simulink model "Start"  (R2016b)
settings: Solver=FixedStepDiscrete  StartTime=0.0  StopTime=60  FixedStep=0.0001  MaxStep=0.001  RelTol=1e-3
undefined symbols (not defined in the file): kat
libraries: simulink x9, microdaq_lib x5
settings Model: SimulationMode=external  ExtModeTrigDuration=10000  Creator=student  LastModifiedBy=barte
settings DataIOCC: MaxDataPoints=100000  SaveFormat=Array
settings DebuggingCC: ParameterTunabilityLossMsg=error
settings HardwareCC: ProdBitPerLong=40  ProdBitPerPointer=32  ProdBitPerSizeT=32  ProdBitPerPtrDiffT=32  ProdLargestAtomicInteger=Integer  ProdLargestAtomicFloat=None  ProdWordSize=32  ProdHWDeviceType=Texas Instruments->C6000
settings RTWCC: SystemTargetFile=microdaq.tlc  TemplateMakefile=microdaq.tmf  PostCodeGenCommand=microdaq_postcodegen(buildInfo)  Description=MicroDAQ Real-Time Measurement System  GenerateReport=on  IncludeHyperlinkInReport=on  LaunchReport=on  GenerateTraceInfo=on  GenerateTraceReport=on  GenerateTraceReportSl=on  GenerateTraceReportSf=on  GenerateTraceReportEml=on
settings CodeAppCC: ForceParamTrailComments=on  IgnoreCustomStorageClasses=off  OperatorAnnotations=on  SimulinkDataObjDesc=on  SFDataObjDesc=on  MATLABFcnDesc=on  InsertBlockDesc=on  MATLABSourceComments=on
settings STFCustomTargetCC: TargetLangStandard=C99 (ISO)  CombineOutputUpdateFcns=on  ERTCustomFileBanners=on  SupportNonInlinedSFcns=off  RemoveResetFunc=on  MATLABClassNameForMDSCustomization=Simulink.SoftwareTarget.ERTCustomization  GRTInterface=off  SystemTargetFile=microdaq.tlc
settings ERTTargetCC: TargetLangStandard=C99 (ISO)  ParMdlRefBuildCompliant=off  CompOptLevelCompliant=off  ConcurrentExecutionCompliant=off  ERTFirstTimeCompliant=off  SupportContinuousTime=on  ModelStepFunctionPrototypeControlCompliant=off  CPPClassGenCompliant=off  UseToolchainInfoCompliant=off  ExtMode=on  ExtModeStaticAlloc=on  ExtModeStaticAllocSize=1085760  ExtModeMexArgs=getpref('microdaq','TargetIP') 1 4344  ERTCustomFileTemplate=microdaq_main.tlc

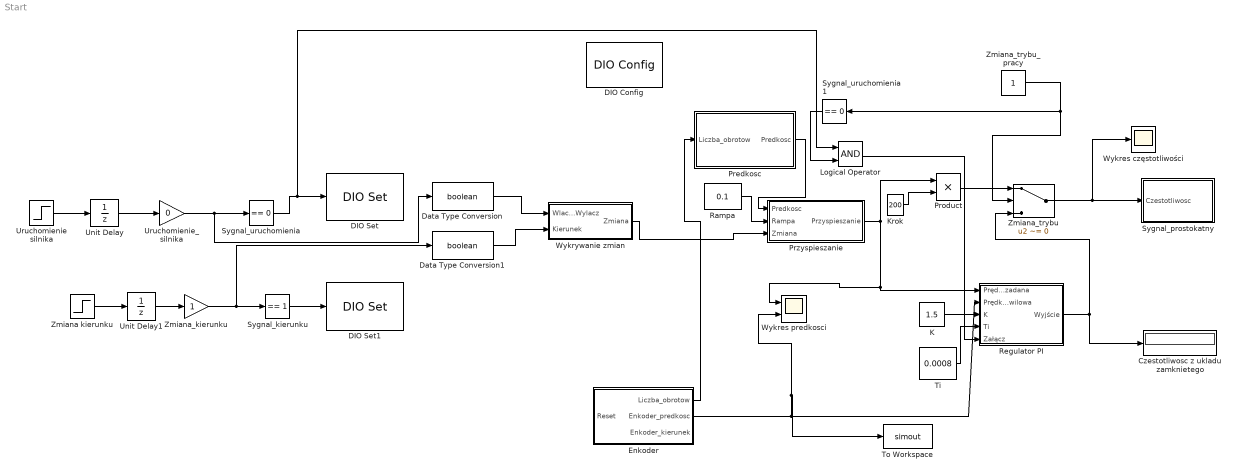
== system Start ==
  "Czestotliwosc z ukladu zamknietego " : Display
  DIO Config : microdaq_lib/Digital/DIO Config  SParameter1=Enable  SParameter2=Enable  SParameter3=Enable  SParameter4=Enable  SParameter5=Enable  SParameter6=Enable  SParameter7=Input  SParameter8=Output  SParameter9=Output  SParameter10=Input
  DIO Set : microdaq_lib/Digital/DIO Set  pDIOpin=DIO21  pDIOdir=ones([1 1 ])  pDIOinitValue=Low  pDIOtermValue=High  SampleTime=-1
  DIO Set1 : microdaq_lib/Digital/DIO Set  pDIOpin=DIO19  pDIOdir=ones([1 1 ])  pDIOinitValue=Low  pDIOtermValue=High  SampleTime=-1
  Data Type Conversion : DataTypeConversion  OutDataTypeStr=boolean
  Data Type Conversion1 : DataTypeConversion  OutDataTypeStr=boolean
  Enkoder : Subsystem
  "K " : Constant  Value=1.5
  "Krok " : Constant  Value=200
  Logical Operator : Logic  AllPortsSameDT=off  OutDataTypeStr=boolean
  Predkosc : Subsystem
  Product : Product  OutDataTypeStr=uint32  RndMeth=Round
  Przyspieszanie : Subsystem
  Rampa : Constant  Value=0.1  OutDataTypeStr=double
  Regulator PI : Subsystem
  Sygnal_kierunku : simulink/Logic and Bit Operations/Compare To Constant  relop===  const=1  OutDataTypeStr=uint8
  Sygnal_prostokatny : Subsystem
  Sygnal_uruchomienia : simulink/Logic and Bit Operations/Compare To Constant  relop===  const=0  OutDataTypeStr=uint8
  Sygnal_uruchomienia1 : simulink/Logic and Bit Operations/Compare To Constant  relop===  const=0  OutDataTypeStr=uint8
  Ti : Constant  Value=0.0008
  To Workspace : ToWorkspace  VariableName=simout  SaveFormat=Timeseries  SampleTime=0.01
  Unit Delay : UnitDelay  SampleTime=-1
  Unit Delay1 : UnitDelay  SampleTime=-1
  Uruchomienie silnika : Step  Time=0.01  SampleTime=0.01
  Uruchomienie_silnika : Gain  Gain=0
  Wykres częstotliwości : Scope
  Wykres predkosci : Scope  NumInputPorts=2
  Wykrywanie zmian : Subsystem
  Zmiana kierunku : Step  Time=0.01  SampleTime=0.01
  Zmiana_kierunku : Gain
  Zmiana_trybu : Switch  Criteria=u2 ~= 0
  Zmiana_trybu_pracy : Constant
  wires:
  Wykrywanie zmian/1(Zmiana) -> Przyspieszanie/3(Zmiana)
  "Krok "/1 -> Product/2
  Rampa/1 -> Przyspieszanie/2(Rampa)
  Data Type Conversion1/1 -> Wykrywanie zmian/2(Kierunek)
  Zmiana kierunku/1 -> Unit Delay1/1
  Uruchomienie silnika/1 -> Unit Delay/1
  Sygnal_kierunku/1 -> DIO Set1/1
  Sygnal_uruchomienia/1 -> Logical Operator/1, DIO Set/1
  Unit Delay/1 -> Uruchomienie_silnika/1
  Unit Delay1/1 -> Zmiana_kierunku/1
  "K "/1 -> Regulator PI/3(K)
  Ti/1 -> Regulator PI/4(Ti)
  Uruchomienie_silnika/1 -> Sygnal_uruchomienia/1, Data Type Conversion/1
  Zmiana_trybu_pracy/1 -> Sygnal_uruchomienia1/1, Zmiana_trybu/2
  Regulator PI/1(Wyjście) -> "Czestotliwosc z ukladu zamknietego "/1, Zmiana_trybu/3
  Zmiana_kierunku/1 -> Data Type Conversion1/1, Sygnal_kierunku/1
  Zmiana_trybu/1 -> Wykres częstotliwości/1, Sygnal_prostokatny/1(Czestotliwosc)
  Przyspieszanie/1(Przyspieszanie) -> Wykres predkosci/1, Regulator PI/1(Prędkość zadana), Product/1
  Product/1 -> Zmiana_trybu/1
  Predkosc/1(Predkosc) -> Przyspieszanie/1(Predkosc)
  Enkoder/1(Liczba_obrotow) -> Predkosc/1(Liczba_obrotow)
  Enkoder/2(Enkoder_predkosc) -> To Workspace/1, Wykres predkosci/2, Regulator PI/2(Prędkość chwilowa)
  Data Type Conversion/1 -> Wykrywanie zmian/1(Wlacz/Wylacz)
  Sygnal_uruchomienia1/1 -> Logical Operator/2
  Logical Operator/1 -> Regulator PI/5(Załącz)

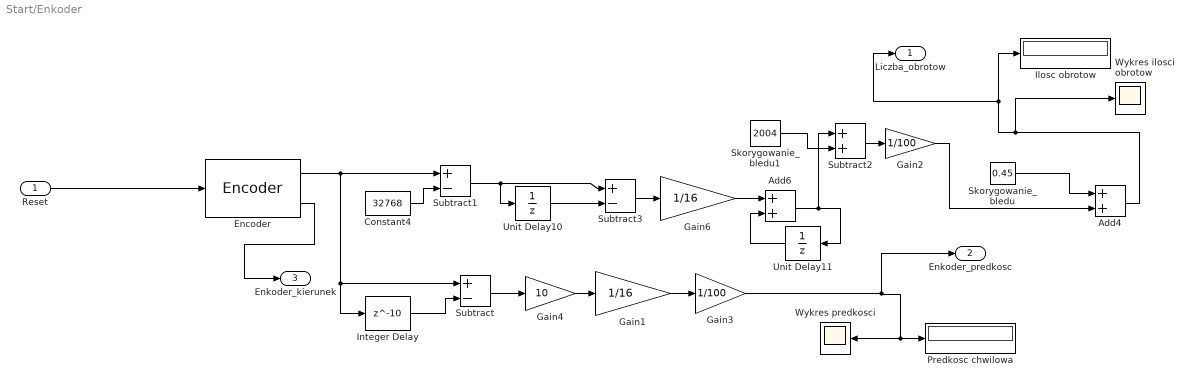
== system Start/Enkoder ==
  Reset : Inport
  Add4 : Sum
  Add6 : Sum  OutDataTypeStr=int32
  Constant4 : Constant  Value=32768  OutDataTypeStr=uint16
  Encoder : microdaq_lib/Motor Control/Encoder  pChannel=ENC1  SampleTime=0.01
  Gain1 : Gain  Gain=1/16  ParamDataTypeStr=double  OutDataTypeStr=int16  RndMeth=Round
  Gain2 : Gain  Gain=1/100
  Gain3 : Gain  Gain=1/100  ParamDataTypeStr=double  OutDataTypeStr=int16  RndMeth=Round
  Gain4 : Gain  Gain=10  ParamDataTypeStr=double  OutDataTypeStr=int16  RndMeth=Round
  Gain6 : Gain  Gain=1/16  ParamDataTypeStr=double  OutDataTypeStr=int16  RndMeth=Round
  "Ilosc obrotow " : Display
      settings: Decimation=2
  Integer Delay : Delay  DelayLength=10
  "Predkosc chwilowa " : Display
      settings: Decimation=2
  Skorygowanie_bledu : Constant  Value=0.45  OutDataTypeStr=double
  Skorygowanie_bledu1 : Constant  Value=2004
  Subtract : Sum  Inputs=+-  AccumDataTypeStr=int16  OutDataTypeStr=uint16  RndMeth=Round
  Subtract1 : Sum  Inputs=+-  OutDataTypeStr=int16
  Subtract2 : Sum  OutDataTypeStr=int16
  Subtract3 : Sum  Inputs=+-  OutDataTypeStr=int16
  Unit Delay10 : UnitDelay  SampleTime=0.01
  Unit Delay11 : UnitDelay  SampleTime=0.01
  "Wykres ilosci obrotow " : Scope
  Wykres predkosci : Scope
  Liczba_obrotow : Outport
  Enkoder_predkosc : Outport  Port=2
  Enkoder_kierunek : Outport  Port=3
  wires:
  Encoder/2 -> Enkoder_kierunek/1
  Reset/1 -> Encoder/1
  Encoder/1 -> Subtract/1, Integer Delay/1, Subtract1/1
  Unit Delay11/1 -> Add6/2
  Unit Delay10/1 -> Subtract3/2
  Subtract3/1 -> Gain6/1
  Integer Delay/1 -> Subtract/2
  Constant4/1 -> Subtract1/2
  Gain6/1 -> Add6/1
  Subtract1/1 -> Subtract3/1, Unit Delay10/1
  Skorygowanie_bledu1/1 -> Subtract2/2
  Add6/1 -> Unit Delay11/1, Subtract2/1
  Subtract2/1 -> Gain2/1
  Skorygowanie_bledu/1 -> Add4/1
  Gain2/1 -> Add4/2
  Add4/1 -> Liczba_obrotow/1, "Ilosc obrotow "/1, "Wykres ilosci obrotow "/1
  Gain1/1 -> Gain3/1
  Subtract/1 -> Gain4/1
  Gain3/1 -> Enkoder_predkosc/1, "Predkosc chwilowa "/1, Wykres predkosci/1
  Gain4/1 -> Gain1/1

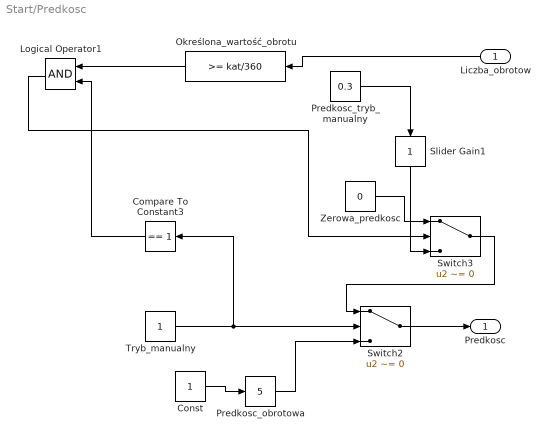
== system Start/Predkosc ==
  Liczba_obrotow : Inport
  Compare To Constant3 : simulink/Logic and Bit Operations/Compare To Constant  relop===  const=1  OutDataTypeStr=uint8
  Const : Constant
  Logical Operator1 : Logic  AllPortsSameDT=off  OutDataTypeStr=boolean
  Określona_wartość_obrotu : simulink/Logic and Bit Operations/Compare To Constant  relop=>=  const=kat/360  OutDataTypeStr=uint8
  Predkosc_obrotowa : simulink/Math Operations/Slider Gain  low=0  gain=5  high=10
  Predkosc_tryb_manualny : Constant  Value=0.3
  Slider Gain1 : simulink/Math Operations/Slider Gain  low=0  gain=1  high=1
  Switch2 : Switch  Criteria=u2 ~= 0  Threshold=1  OutDataTypeStr=double
  Switch3 : Switch  Criteria=u2 ~= 0  Threshold=1  OutDataTypeStr=double
  Tryb_manualny : Constant
  Zerowa_predkosc : Constant  Value=0
  Predkosc : Outport
  wires:
  Slider Gain1/1 -> Switch3/3
  Predkosc_tryb_manualny/1 -> Slider Gain1/1
  Tryb_manualny/1 -> Switch2/2, Compare To Constant3/1
  Compare To Constant3/1 -> Logical Operator1/2
  Switch2/1 -> Predkosc/1
  Określona_wartość_obrotu/1 -> Logical Operator1/1
  Zerowa_predkosc/1 -> Switch3/1
  Logical Operator1/1 -> Switch3/2
  Const/1 -> Predkosc_obrotowa/1
  Predkosc_obrotowa/1 -> Switch2/3
  Switch3/1 -> Switch2/1
  Liczba_obrotow/1 -> Określona_wartość_obrotu/1

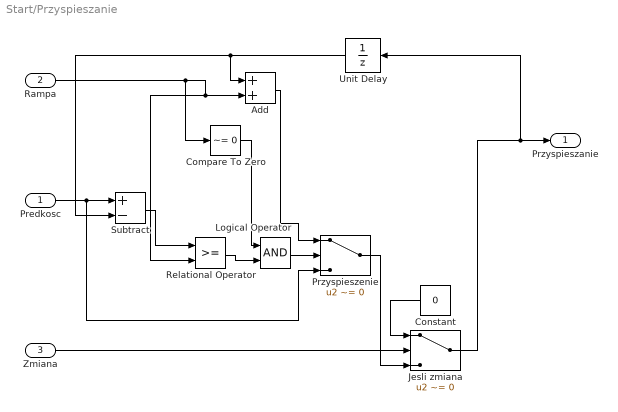
== system Start/Przyspieszanie ==
  Predkosc : Inport
  Rampa : Inport  Port=2  SampleTime=0.01
  Zmiana : Inport  Port=3  OutDataTypeStr=boolean
  Add : Sum  OutDataTypeStr=double
  Compare To Zero : simulink/Logic and Bit Operations/Compare To Zero  relop=~=  OutDataTypeStr=boolean
  Constant : Constant  Value=0  OutDataTypeStr=uint16
  Jesli zmiana : Switch  Criteria=u2 ~= 0  OutDataTypeStr=double
  Logical Operator : Logic  AllPortsSameDT=off  OutDataTypeStr=boolean
  Przyspieszenie : Switch  Criteria=u2 ~= 0  OutDataTypeStr=double
  Relational Operator : RelationalOperator  OutDataTypeStr=boolean  RndMeth=Nearest
  Subtract : Sum  Inputs=+-  OutDataTypeStr=double
  Unit Delay : UnitDelay  SampleTime=0.01
  Przyspieszanie : Outport  OutDataTypeStr=double
  wires:
  Rampa/1 -> Relational Operator/2, Add/2, Compare To Zero/1
  Unit Delay/1 -> Add/1, Subtract/2
  Subtract/1 -> Relational Operator/1
  Add/1 -> Przyspieszenie/1
  Zmiana/1 -> Jesli zmiana/2
  Constant/1 -> Jesli zmiana/1
  Przyspieszenie/1 -> Jesli zmiana/3
  Jesli zmiana/1 -> Przyspieszanie/1, Unit Delay/1
  Predkosc/1 -> Przyspieszenie/3, Subtract/1
  Relational Operator/1 -> Logical Operator/2
  Compare To Zero/1 -> Logical Operator/1
  Logical Operator/1 -> Przyspieszenie/2

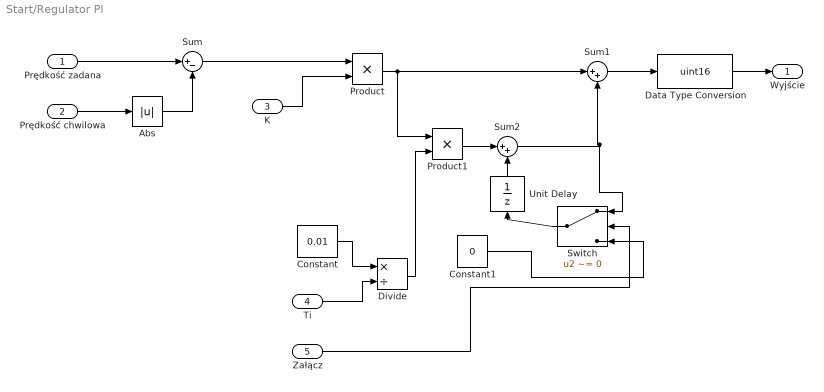
== system Start/Regulator PI ==
  Prędkość zadana : Inport
  Prędkość chwilowa : Inport  Port=2
  K : Inport  Port=3
  Ti : Inport  Port=4
  Załącz : Inport  Port=5
  Abs : Abs
  Constant : Constant  Value=0.01
  Constant1 : Constant  Value=0
  Data Type Conversion : DataTypeConversion  OutDataTypeStr=uint16
  Divide : Product  Inputs=*/
  Product : Product  RndMeth=Zero
  Product1 : Product  RndMeth=Zero
  Sum : Sum  Inputs=|+-  AccumDataTypeStr=double  OutDataTypeStr=double
  Sum1 : Sum  Inputs=|++
  Sum2 : Sum  Inputs=|++
  Switch : Switch  Criteria=u2 ~= 0
  Unit Delay : UnitDelay  SampleTime=0.01
  Wyjście : Outport
  wires:
  Prędkość zadana/1 -> Sum/1
  Constant/1 -> Divide/1
  Ti/1 -> Divide/2
  Divide/1 -> Product1/2
  Product1/1 -> Sum2/1
  Data Type Conversion/1 -> Wyjście/1
  Sum/1 -> Product/1
  K/1 -> Product/2
  Product/1 -> Sum1/1, Product1/1
  Abs/1 -> Sum/2
  Sum1/1 -> Data Type Conversion/1
  Prędkość chwilowa/1 -> Abs/1
  Unit Delay/1 -> Sum2/2
  Switch/1 -> Unit Delay/1
  Sum2/1 -> Switch/1, Sum1/2
  Załącz/1 -> Switch/2
  Constant1/1 -> Switch/3

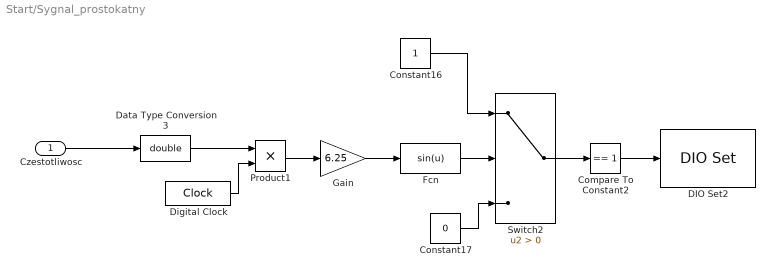
== system Start/Sygnal_prostokatny ==
  Czestotliwosc : Inport
  Compare To Constant2 : simulink/Logic and Bit Operations/Compare To Constant  relop===  const=1  OutDataTypeStr=uint8
  Constant16 : Constant
  Constant17 : Constant  Value=0
  DIO Set2 : microdaq_lib/Digital/DIO Set  pDIOpin=DIO17  pDIOdir=ones([1 1 ])  pDIOinitValue=Low  pDIOtermValue=High  SampleTime=-1
  Data Type Conversion3 : DataTypeConversion  OutDataTypeStr=double
  Digital Clock : DigitalClock  SampleTime=0.0001
  Fcn : Fcn  Expr=sin(u)
  Gain : Gain  Gain=6.25
  Product1 : Product
  Switch2 : Switch  Criteria=u2 > Threshold
  wires:
  Czestotliwosc/1 -> Data Type Conversion3/1
  Data Type Conversion3/1 -> Product1/1
  Fcn/1 -> Switch2/2
  Constant17/1 -> Switch2/3
  Constant16/1 -> Switch2/1
  Gain/1 -> Fcn/1
  Product1/1 -> Gain/1
  Compare To Constant2/1 -> DIO Set2/1
  Switch2/1 -> Compare To Constant2/1
  Digital Clock/1 -> Product1/2

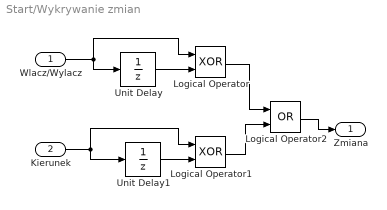
== system Start/Wykrywanie zmian ==
  Wlacz/Wylacz : Inport  OutDataTypeStr=boolean
  Kierunek : Inport  Port=2  OutDataTypeStr=boolean
  Logical Operator : Logic  Operator=XOR  AllPortsSameDT=off  OutDataTypeStr=boolean
  Logical Operator1 : Logic  Operator=XOR  AllPortsSameDT=off  OutDataTypeStr=boolean
  Logical Operator2 : Logic  Operator=OR  AllPortsSameDT=off  OutDataTypeStr=boolean
  Unit Delay : UnitDelay  SampleTime=0.01
  Unit Delay1 : UnitDelay  SampleTime=0.01
  Zmiana : Outport  OutDataTypeStr=boolean
  wires:
  Wlacz/Wylacz/1 -> Logical Operator/1, Unit Delay/1
  Kierunek/1 -> Logical Operator1/1, Unit Delay1/1
  Logical Operator2/1 -> Zmiana/1
  Unit Delay1/1 -> Logical Operator1/2
  Unit Delay/1 -> Logical Operator/2
  Logical Operator1/1 -> Logical Operator2/2
  Logical Operator/1 -> Logical Operator2/1
